simulink model "dead_time_sim"  (R2024b)
settings: Solver=VariableStepAuto  StartTime=0.0  StopTime=10.0  RelTol=1e-3
values from neighbouring files (symbols this model uses):
  A = [-a_(2:end)', [1; 0]]    [atv5.m]    (also in example1_1.m)
  B = b(2:3)'    [atv5.m]    (also in example1_1.m)
  D = -a_(2:end)'    [atv5.m]    (also in example1_1.m)
  H = [1, 0]    [atv5.m]    (also in example1_1.m)
  Kr = sum(K)    [atv5.m]    (also in example1_1.m)
undefined symbols (not defined in the file or in its folder): d
libraries: cstblocks x2
settings Model: Creator=room2  LastModifiedBy=room2

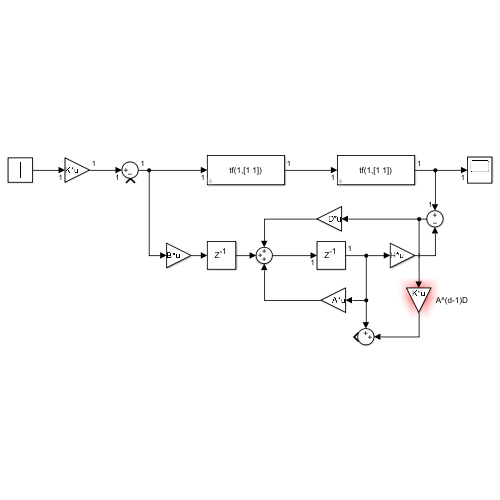
[thumbnail: Simulink's stored preview of the top-level diagram]
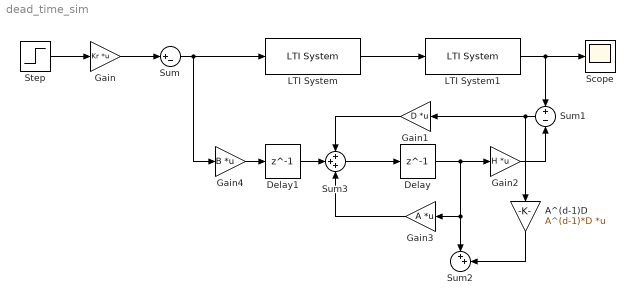
== system dead_time_sim ==
  A^(d-1)D : Gain  Gain=A^(d-1)*D  Multiplication=Matrix(K*u)
  Delay : Delay  DelayLength=1
  Delay1 : Delay  DelayLength=1
  Gain : Gain  Gain=Kr  Multiplication=Matrix(K*u)
  Gain1 : Gain  Gain=D  Multiplication=Matrix(K*u)
  Gain2 : Gain  Gain=H  Multiplication=Matrix(K*u)
  Gain3 : Gain  Gain=A  Multiplication=Matrix(K*u)
  Gain4 : Gain  Gain=B  Multiplication=Matrix(K*u)
  LTI System : cstblocks/LTI System  sys=tf(1,[1 1])  IC=[]  PadeOrder=0
  LTI System1 : cstblocks/LTI System  sys=tf(1,[1 1])  IC=[]  PadeOrder=0
  Scope : Scope
  Step : Step  SampleTime=0
  Sum : Sum  Inputs=|+-
  Sum1 : Sum  Inputs=+-
  Sum2 : Sum  Inputs=++|
  Sum3 : Sum  Inputs=+++
  wires:
  Step/1 -> Gain/1
  Gain/1 -> Sum/1
  Sum/1 -> Gain4/1, LTI System/1
  LTI System/1 -> LTI System1/1
  LTI System1/1 -> Scope/1, Sum1/1
  Sum1/1 -> A^(d-1)D/1, Gain1/1
  Gain2/1 -> Sum1/2
  Delay/1 -> Gain2/1, Sum2/1, Gain3/1
  A^(d-1)D/1 -> Sum2/2
  Gain1/1 -> Sum3/1
  Gain3/1 -> Sum3/3
  Sum3/1 -> Delay/1
  Gain4/1 -> Delay1/1
  Delay1/1 -> Sum3/2
